simulink model "chua_sim"  (R2023b)
settings: Solver=ode45  StartTime=0.0  StopTime=Tfin  RelTol=1e-3  EnableMultiTasking=on
undefined symbols (not defined in the file or in its folder): chua_circuit, u_bar, x0, x0_p
settings Model: Creator=s329152  LastModifiedBy=Msi
settings SolverCC: AlgebraicLoopSolver=TrustRegion
settings DataIOCC: LimitDataPoints=on  SaveFormat=Array  ReturnWorkspaceOutputs=off
settings OptimizationCC: LifeSpan=inf
settings DebuggingCC: SolverPrmCheckMsg=warning  UnconnectedInputMsg=warning  UnconnectedOutputMsg=warning  UnconnectedLineMsg=warning  SFUnexpectedBacktrackingDiag=warning  SFNoUnconditionalDefaultTransitionDiag=warning  SFExecutionAtInitializationDiag=none  ArithmeticOperatorsInVariantConditions=warning
settings HardwareCC: ProdBitPerPointer=32  ProdBitPerSizeT=32  ProdBitPerPtrDiffT=32  ProdLargestAtomicFloat=None  ProdIntDivRoundTo=Undefined  ProdEndianess=Unspecified  ProdWordSize=32  ProdHWDeviceType=32-bit Generic
settings ModelReferenceCC: PropagateSignalLabelsOutOfModel=off
settings SFSimCC: SimUseLocalCustomCode=off  CustomCodeUndefinedFunction=UseInterfaceOnly
settings RTWCC: RTWUseLocalCustomCode=off
settings CodeAppCC: StateflowObjectComments=on
settings GRTTargetCC: TargetLangStandard=C89/C90 (ANSI)
settings ConfigComp: CovMetricSettings=dw  CovSaveCumulativeToWorkspaceVar=on  CovSaveSingleToWorkspaceVar=on  CovExternalEMLEnable=off  CovSFcnEnable=off

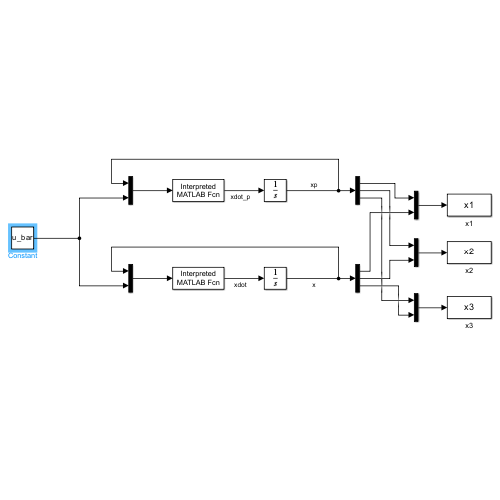
[thumbnail: Simulink's stored preview of the top-level diagram]
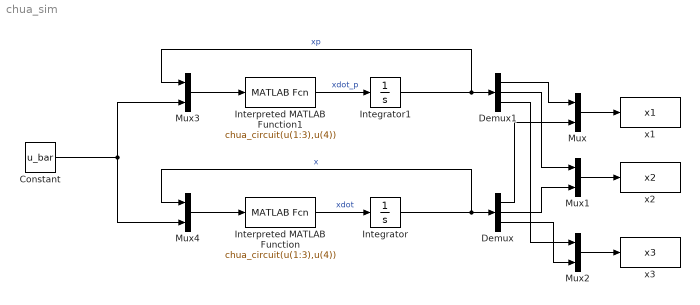
== system chua_sim ==
  Constant : Constant  Value=u_bar  SampleTime=0.1
  Demux : Demux  Outputs=3
  Demux1 : Demux  Outputs=3
  Integrator : Integrator  InitialCondition=x0
  Integrator1 : Integrator  InitialCondition=x0_p
  Interpreted MATLAB Function : MATLABFcn  MATLABFcn=chua_circuit(u(1:3),u(4))
  Interpreted MATLAB Function1 : MATLABFcn  MATLABFcn=chua_circuit(u(1:3),u(4))
  Mux{,1..4} (5 alike) : Mux  Inputs=2
  x1 : ToWorkspace  VariableName=x1  SampleTime=0.1
  x2 : ToWorkspace  VariableName=x2  SampleTime=0.1
  "x3 " : ToWorkspace  VariableName=x3  SampleTime=0.1
  wires:
  Interpreted MATLAB Function/1 -> Integrator/1  "xdot"
  Integrator/1 -> Mux4/1, Demux/1  "x"
  Interpreted MATLAB Function1/1 -> Integrator1/1  "xdot_p"
  Integrator1/1 -> Mux3/1, Demux1/1  "xp"
  Demux1/1 -> Mux/1
  Demux/1 -> Mux/2
  Mux/1 -> x1/1
  Demux/2 -> Mux1/2
  Demux1/2 -> Mux1/1
  Mux1/1 -> x2/1
  Demux1/3 -> Mux2/1
  Demux/3 -> Mux2/2
  Mux2/1 -> "x3 "/1
  Constant/1 -> Mux4/2, Mux3/2
  Mux3/1 -> Interpreted MATLAB Function1/1
  Mux4/1 -> Interpreted MATLAB Function/1
